simulink model "rths_tp82dd61fb_5441_4646_94f0_6aae3426dff9"  (R2025b)
settings: Solver=ode4  StartTime=0.0  StopTime=40  FixedStep=dt  RelTol=1e-3
model workspace (MAT data in the model file):
  A1 = [0 0 0 0 0 0 0 0 0 0 0 0 ... (900 elements, 30x30)]
  A2 = [0  0  0  0  0  0  1  0  0  0  0  0; 0  0  0  0  0  0  0  1  0  0  0  0; 0  0  0  0  0  0  0  0  1  0  0  0; 0  0  0  0  0  0  0  0  0  1  0  0; 0  0  0  0  0  0  0  0  0  0  1  0; 0  0  0  0  0  0  0  0  0  0  0  1; -11321.1034388  6271.05467548  -1128.48907858  10.995990455  470.039389184  19.2527594147  -16.2888377097  8.29248155512  -1.49224896824  0.0145404645226  0.621553018861  0.0254587402907; 6271.05467548  -8717.09362481  3966.53742016  -478.296158144  8.25676895975  439.790639314  8.29248155512  -12.8454450957  5.24512065298  -0.632471294629  0.0109182757681  0.581553814048; -1128.48907858  3966.53742016  -3080.31145452  -6.8676059751  -489.292148599  -454.915014249  -1.49224896824  5.24512065298  -5.3916889739  -0.00908132663857  -0.647011759152  -0.601553416454; 998.544415132  -43434.0098283  -623.646375453  -48040.5640967  -10069.9090082  17.6940677908  1.32041762876  -57.4346332482  -0.824674051333  -64.8445378234  -13.31586775  0.0233976162517; 42684.2137489  749.796079357  -44432.5542434  -10069.9090082  -48022.8700289  -10105.2971438  56.4431460934  0.991487154861  -58.755050877  -13.31586775  -64.8211402072  -13.3626629825; 1748.34049449  39937.3288393  -41310.7712941  17.6940677908  -10105.2971438  -27829.9698092  2.31190478362  52.810823681  -54.6269848872  0.0233976162517  -13.3626629825  -38.1192118583]
  A3 = [0 0 0 0 0 0 0 0 0 -11216.7436102 6120.49164694 -1250.45258802 ... (324 elements, 18x18)]
  B1 = [0  0  0  0  0  0  0  0  0  0  0  0  0  0  0; 0  0  0  0  0  0  0  0  0  0  0  0  0  0  0; 0  0  0  0  0  0  0  0  0  0  0  0  0  0  0; 0  0  0  0  0  0  0  0  0  0  0  0  0  0  0; 0  0  0  0  0  0  0  0  0  0  0  0  0  0  0; 0  0  0  0  0  0  0  0  0  0  0  0  0  0  0; 0  0  0  0  0  0  0  0  0  0  0  0  0  0  0; 0  0  0  0  0  0  0  0  0  0  0  0  0  0  0; 0  0  0  0  0  0  0  0  0  0  0  0  0  0  0; 0  0  0  0  0  0  0  0  0  0  0  0  0  0  0; 0  0  0  0  0  0  0  0  0  0  0  0  0  0  0; 0  0  0  0  0  0  0  0  0  0  0  0  0  0  0; 0  0  0  0  0  0  0  0  0  0  0  0  0  0  0; 0  0  0  0  0  0  0  0  0  0  0  0  0  0  0; 0  0  0  0  0  0  0  0  0  0  0  0  0  0  0; 0.000162210458758  0  0  0  0  0  0  0  0  0  0  0  0  0  0; 0  0.0195741403137  0  0  0  0  0  0  0  0  0  0  0  0  0; 0  0  0.0147303099554  0  0  0  0  0  0  0  0  0  0  0  0; 0  0  0  0.0147303099554  0  0  0  0  0  0  0  0  0  0  0; 0  0  0  0  0.0195741403137  0  0  0  0  0  0  0  0  0  0; 0  0  0  0  0  0.000162210458758  0  0  0  0  0  0  0  0  0; 0  0  0  0  0  0  0.0195741403137  0  0  0  0  0  0  0  0; 0  0  0  0  0  0  0  0.0147303099554  0  0  0  0  0  0  0; 0  0  0  0  0  0  0  0  0.0147303099554  0  0  0  0  0  0; 0  0  0  0  0  0  0  0  0  0.0195741403137  0  0  0  0  0; 0  0  0  0  0  0  0  0  0  0  0.000162210458758  0  0  0  0; 0  0  0  0  0  0  0  0  0  0  0  0.0195741403137  0  0  0; 0  0  0  0  0  0  0  0  0  0  0  0  0.0147303099554  0  0; 0  0  0  0  0  0  0  0  0  0  0  0  0  0.0147303099554  0; 0  0  0  0  0  0  0  0  0  0  0  0  0  0  0.0195741403137]
  B2 = [0  0  0  0  0  0; 0  0  0  0  0  0; 0  0  0  0  0  0; 0  0  0  0  0  0; 0  0  0  0  0  0; 0  0  0  0  0  0; 0.000162210458758  0  0  0  0  0; 0  0.000162210458758  0  0  0  0; 0  0  0.000162210458758  0  0  0; 0  0  0  0.0147303099554  0  0; 0  0  0  0  0.0147303099554  0; 0  0  0  0  0  0.0147303099554]
  B3 = [0  0  0  0  0  0  0  0  0; 0  0  0  0  0  0  0  0  0; 0  0  0  0  0  0  0  0  0; 0  0  0  0  0  0  0  0  0; 0  0  0  0  0  0  0  0  0; 0  0  0  0  0  0  0  0  0; 0  0  0  0  0  0  0  0  0; 0  0  0  0  0  0  0  0  0; 0  0  0  0  0  0  0  0  0; 0.000159186201117  -2.54024240345e-06  4.65575255871e-06  -2.40646746724e-06  8.1196183977e-06  4.37381616231e-06  0.000302935336269  0.00126264599362  0.00156203975266; -2.54024240345e-06  0.000154107993859  4.88016101925e-06  -1.54311353769e-05  6.77864041829e-06  6.25450457057e-06  -0.000459326699367  -0.00191449113814  -0.0023684479094; 4.65575255871e-06  4.88016101925e-06  0.000154885583422  5.88289993993e-06  -1.24931676457e-05  -7.15255052644e-06  0.000293964918962  0.00122525695339  0.0015157851671; -2.40646746724e-06  -1.54311353769e-05  5.88289993993e-06  0.014680380812  1.08842148256e-05  1.49205088267e-05  0.001698259817  0.00213312637172  0.0011075391107; 8.1196183977e-06  6.77864041829e-06  -1.24931676457e-05  1.08842148256e-05  0.0146962651234  -1.84930265115e-05  -0.00411085573378  -0.00486398973958  -0.00221765410407; 4.37381616231e-06  6.25450457057e-06  -7.15255052644e-06  1.49205088267e-05  -1.84930265115e-05  0.0147185175842  0.00845575577146  0.00974441342285  0.0041586471669; 0.000302935336269  -0.000459326699367  0.000293964918962  0.001698259817  -0.00411085573378  0.00845575577146  1.00869498175  0.0176088889684  0.016014507749; 0.00126264599362  -0.00191449113814  0.00122525695339  0.00213312637172  -0.00486398973958  0.00974441342285  0.0176088889684  1.05175826224  0.057330972257; 0.00156203975266  -0.0023684479094  0.0015157851671  0.0011075391107  -0.00221765410407  0.0041586471669  0.016014507749  0.057330972257  1.06800860627]
  C1 = [1  0  0  0  0  0  0  0  0  0  0  0  0  0  0  0  0  0  0  0  0  0  0  0  0  0  0  0  0  0; 0  0  0  0  0  1  0  0  0  0  0  0  0  0  0  0  0  0  0  0  0  0  0  0  0  0  0  0  0  0; 0  0  0  0  0  0  0  0  0  0  1  0  0  0  0  0  0  0  0  0  0  0  0  0  0  0  0  0  0  0]
  C2 = [1  0  0  0  0  0  0  0  0  0  0  0; 0  1  0  0  0  0  0  0  0  0  0  0; 0  0  1  0  0  0  0  0  0  0  0  0]
  C3 = [1  0  0  0  0  0  0  0  0  0  0  0  0  0  0  0  0  0; 0  1  0  0  0  0  0  0  0  0  0  0  0  0  0  0  0  0; 0  0  1  0  0  0  0  0  0  0  0  0  0  0  0  0  0  0]
  D1 = [0  0  0  0  0  0  0  0  0  0  0  0  0  0  0; 0  0  0  0  0  0  0  0  0  0  0  0  0  0  0; 0  0  0  0  0  0  0  0  0  0  0  0  0  0  0]
  D2 = [0  0  0  0  0  0; 0  0  0  0  0  0; 0  0  0  0  0  0]
  D3 = [0  0  0  0  0  0  0  0  0; 0  0  0  0  0  0  0  0  0; 0  0  0  0  0  0  0  0  0]
  cb_force = [6164.83060128; 6164.83060128; 6164.83060128; 0; 0; 0; 0; 0; 0]
  dt = 0.0009765625
  excitation_input = [0 0.0009765625 0.001953125 0.0029296875 0.00390625 0.0048828125 0.005859375 0.0068359375 0.0078125 0.0087890625 0.009765625 0.0107421875 ... (81922 elements, 40961x2)]
  full_force = [6164.83060128; 0; 0; 0; 0; 6164.83060128; 0; 0; 0; 0; 6164.83060128; 0; 0; 0; 0]
  guyan_force = [6164.83060128; 6164.83060128; 6164.83060128; 0; 0; 0]
settings Model: Creator=lenovo  LastModifiedBy=lenovo
settings DataIOCC: SaveOutput=off  SignalLogging=off  SaveTime=off

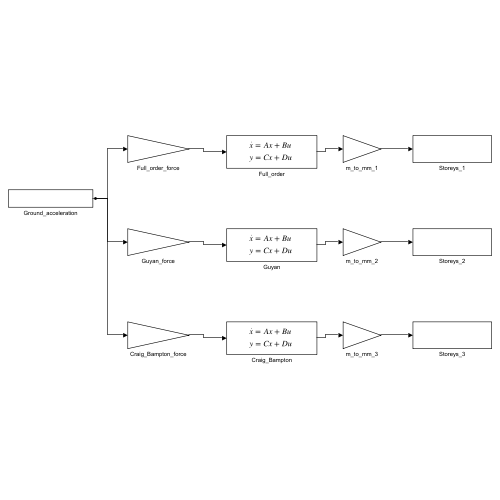
[thumbnail: Simulink's stored preview of the top-level diagram]
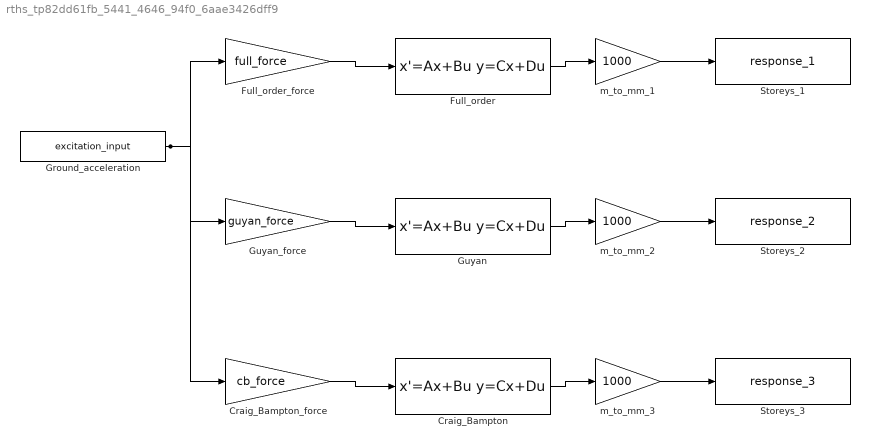
== system rths_tp82dd61fb_5441_4646_94f0_6aae3426dff9 ==
  Craig_Bampton : StateSpace  A=A3  B=B3  C=C3  D=D3  InitialCondition=0
  Craig_Bampton_force : Gain  Gain=cb_force
  Full_order : StateSpace  A=A1  B=B1  C=C1  D=D1  InitialCondition=0
  Full_order_force : Gain  Gain=full_force
  Ground_acceleration : FromWorkspace  VariableName=excitation_input  OutputAfterFinalValue=Holding final value
  Guyan : StateSpace  A=A2  B=B2  C=C2  D=D2  InitialCondition=0
  Guyan_force : Gain  Gain=guyan_force
  Storeys_1 : ToWorkspace  VariableName=response_1  SaveFormat=Timeseries  SampleTime=-1
  Storeys_2 : ToWorkspace  VariableName=response_2  SaveFormat=Timeseries  SampleTime=-1
  Storeys_3 : ToWorkspace  VariableName=response_3  SaveFormat=Timeseries  SampleTime=-1
  m_to_mm_1 : Gain  Gain=1000
  m_to_mm_2 : Gain  Gain=1000
  m_to_mm_3 : Gain  Gain=1000
  wires:
  Ground_acceleration/1 -> Full_order_force/1, Guyan_force/1, Craig_Bampton_force/1
  Full_order_force/1 -> Full_order/1
  Full_order/1 -> m_to_mm_1/1
  m_to_mm_1/1 -> Storeys_1/1
  Guyan_force/1 -> Guyan/1
  Guyan/1 -> m_to_mm_2/1
  m_to_mm_2/1 -> Storeys_2/1
  Craig_Bampton_force/1 -> Craig_Bampton/1
  Craig_Bampton/1 -> m_to_mm_3/1
  m_to_mm_3/1 -> Storeys_3/1
